simulink model "21-E"  (R2014a)
settings: Solver=FixedStepDiscrete  StartTime=0.0  StopTime=10.0  FixedStep=0.0005  RelTol=1e-3
undefined symbols (not defined in the file): add_k1_100, add_k2_100, ADDspeed, cal_acc_div, cal_acc_flo_add, cal_acc_min, cal_an_div, cal_an_min, cal_bre_div, cal_bre_en_add, cal_bre_flo_add, cal_bre_min, cal_conf_off, cal_conf_on, controller, ecucoder_acal, enres_on_add, enres_per_add
libraries: simulink x165, ec55xxlib x29
(part 4 of 6)

== system 21-E/ECU_can/ECU_sig1/yaw_r ==
  yaw_r : Inport
  Constant{1..2,4..8} (7 alike) : Constant  Value=0  OutDataTypeStr=uint8  SampleTime=-1
  yaw_rABS : Abs
  yaw_rCS : ArithShift  BitShiftNumber=-8
  yaw_rConS : Constant  OutDataTypeStr=single
  yaw_rCosR : Constant  Value=0  OutDataTypeStr=uint8
  yaw_rROP : RelationalOperator  Operator=<  OutDataTypeStr=boolean
  yaw_rRon : Rounding  Operator=round
  yaw_rSW : Switch  Criteria=u2 ~= 0
  yaw_r_1sat : Saturate  UpperLimit=255  LowerLimit=0
  yaw_r_Convert : DataTypeConversion  OutDataTypeStr=uint8
  yaw_r_Convert1 : DataTypeConversion  OutDataTypeStr=uint32
  yaw_r_D : Product  Inputs=*/
  yaw_r_F : Constant  OutDataTypeStr=single
  yaw_r_L : simulink/Logic and Bit Operations/Bitwise Operator  logicop=AND  UseBitMask=on  BitMask=255  BitMaskRealWorld=Stored Integer
  yaw_r_O : Constant  Value=0  OutDataTypeStr=single
  yaw_r_S : ArithShift
  yaw_r_sat : Saturate  UpperLimit=255  LowerLimit=0
  yaw_r_st : Sum  Inputs=+-
  yaw_rsubcon : Sum  Inputs=+-
  output1 : Outport
  output2 : Outport  Port=2
  output3 : Outport  Port=3
  output4 : Outport  Port=4
  output5 : Outport  Port=5
  output6 : Outport  Port=6
  output7 : Outport  Port=7
  output8 : Outport  Port=8
  wires:
  Constant8/1 -> output8/1
  Constant7/1 -> output7/1
  Constant6/1 -> output6/1
  Constant5/1 -> output5/1
  Constant4/1 -> output4/1
  Constant2/1 -> output2/1
  Constant1/1 -> output1/1
  yaw_r_Convert/1 -> output3/1
  yaw_r_L/1 -> yaw_r_Convert/1
  yaw_r_Convert1/1 -> yaw_r_L/1
  yaw_r_1sat/1 -> yaw_r_Convert1/1
  yaw_r_S/1 -> yaw_r_1sat/1
  yaw_rSW/1 -> yaw_r_S/1
  yaw_rROP/1 -> yaw_rSW/2
  yaw_rsubcon/1 -> yaw_rSW/1
  yaw_rABS/1 -> yaw_rsubcon/2
  yaw_rCS/1 -> yaw_rsubcon/1
  yaw_rConS/1 -> yaw_rCS/1
  yaw_rCosR/1 -> yaw_rROP/2
  yaw_rRon/1 -> yaw_rSW/3, yaw_rABS/1, yaw_rROP/1
  yaw_r_D/1 -> yaw_rRon/1
  yaw_r_F/1 -> yaw_r_D/2
  yaw_r_st/1 -> yaw_r_D/1
  yaw_r_O/1 -> yaw_r_st/2
  yaw_r_sat/1 -> yaw_r_st/1
  yaw_r/1 -> yaw_r_sat/1

== system 21-E/ECU_can/ECU_speed/v_1L ==
  v_1L : Inport
  BitCov : DataTypeConversion  OutDataTypeStr=uint8
  Constant{3..8} (6 alike) : Constant  Value=0  OutDataTypeStr=uint8
  v_1LCOV : DataTypeConversion  OutDataTypeStr=uint8
  v_1LRon : Rounding  Operator=round
  v_1L_1sat : Saturate  UpperLimit=65535  LowerLimit=0
  v_1L_And : simulink/Logic and Bit Operations/Bitwise Operator  logicop=AND  UseBitMask=off  NumInputPorts=2  BitMask=bin2dec('11011001')  BitMaskRealWorld=Stored Integer
  v_1L_And_C : Constant  Value=255  OutDataTypeStr=uint32
  v_1L_Convert : DataTypeConversion  OutDataTypeStr=uint32
  v_1L_D : Product  Inputs=*/
  v_1L_D1 : Product  Inputs=*/
  v_1L_F : Constant  OutDataTypeStr=single
  v_1L_L : simulink/Logic and Bit Operations/Bitwise Operator  logicop=AND  UseBitMask=on  BitMask=65535  BitMaskRealWorld=Stored Integer
  v_1L_O : Constant  Value=0  OutDataTypeStr=single
  v_1L_S : ArithShift
  v_1L_sat : Saturate  UpperLimit=65535  LowerLimit=0
  v_1L_st : Sum  Inputs=+-
  v_1Loutput2_C : Constant  Value=256
  output1 : Outport
  output2 : Outport  Port=2
  output3 : Outport  Port=3
  output4 : Outport  Port=4
  output5 : Outport  Port=5
  output6 : Outport  Port=6
  output7 : Outport  Port=7
  output8 : Outport  Port=8
  wires:
  Constant8/1 -> output8/1
  Constant7/1 -> output7/1
  Constant6/1 -> output6/1
  Constant5/1 -> output5/1
  Constant4/1 -> output4/1
  Constant3/1 -> output3/1
  BitCov/1 -> output1/1
  v_1L_And/1 -> BitCov/1
  v_1L_And_C/1 -> v_1L_And/2
  v_1LCOV/1 -> output2/1
  v_1L_D1/1 -> v_1LCOV/1
  v_1Loutput2_C/1 -> v_1L_D1/2
  v_1L_L/1 -> v_1L_And/1, v_1L_D1/1
  v_1L_Convert/1 -> v_1L_L/1
  v_1L_1sat/1 -> v_1L_Convert/1
  v_1L_S/1 -> v_1L_1sat/1
  v_1LRon/1 -> v_1L_S/1
  v_1L_D/1 -> v_1LRon/1
  v_1L_F/1 -> v_1L_D/2
  v_1L_st/1 -> v_1L_D/1
  v_1L_O/1 -> v_1L_st/2
  v_1L_sat/1 -> v_1L_st/1
  v_1L/1 -> v_1L_sat/1

== system 21-E/ECU_can/ECU_speed/v_1R ==
  v_1R : Inport
  BitCov : DataTypeConversion  OutDataTypeStr=uint8
  Constant{1..2,5..8} (6 alike) : Constant  Value=0  OutDataTypeStr=uint8
  v_1RCOV : DataTypeConversion  OutDataTypeStr=uint8
  v_1RRon : Rounding  Operator=round
  v_1R_1sat : Saturate  UpperLimit=65535  LowerLimit=0
  v_1R_And : simulink/Logic and Bit Operations/Bitwise Operator  logicop=AND  UseBitMask=off  NumInputPorts=2  BitMask=bin2dec('11011001')  BitMaskRealWorld=Stored Integer
  v_1R_And_C : Constant  Value=255  OutDataTypeStr=uint32
  v_1R_Convert : DataTypeConversion  OutDataTypeStr=uint32
  v_1R_D : Product  Inputs=*/
  v_1R_D1 : Product  Inputs=*/
  v_1R_F : Constant  OutDataTypeStr=single
  v_1R_L : simulink/Logic and Bit Operations/Bitwise Operator  logicop=AND  UseBitMask=on  BitMask=65535  BitMaskRealWorld=Stored Integer
  v_1R_O : Constant  Value=0  OutDataTypeStr=single
  v_1R_S : ArithShift
  v_1R_sat : Saturate  UpperLimit=65535  LowerLimit=0
  v_1R_st : Sum  Inputs=+-
  v_1Routput4_C : Constant  Value=256
  output1 : Outport
  output2 : Outport  Port=2
  output3 : Outport  Port=3
  output4 : Outport  Port=4
  output5 : Outport  Port=5
  output6 : Outport  Port=6
  output7 : Outport  Port=7
  output8 : Outport  Port=8
  wires:
  Constant8/1 -> output8/1
  Constant7/1 -> output7/1
  Constant6/1 -> output6/1
  Constant5/1 -> output5/1
  Constant2/1 -> output2/1
  Constant1/1 -> output1/1
  BitCov/1 -> output3/1
  v_1R_And/1 -> BitCov/1
  v_1R_And_C/1 -> v_1R_And/2
  v_1RCOV/1 -> output4/1
  v_1R_D1/1 -> v_1RCOV/1
  v_1Routput4_C/1 -> v_1R_D1/2
  v_1R_L/1 -> v_1R_And/1, v_1R_D1/1
  v_1R_Convert/1 -> v_1R_L/1
  v_1R_1sat/1 -> v_1R_Convert/1
  v_1R_S/1 -> v_1R_1sat/1
  v_1RRon/1 -> v_1R_S/1
  v_1R_D/1 -> v_1RRon/1
  v_1R_F/1 -> v_1R_D/2
  v_1R_st/1 -> v_1R_D/1
  v_1R_O/1 -> v_1R_st/2
  v_1R_sat/1 -> v_1R_st/1
  v_1R/1 -> v_1R_sat/1

== system 21-E/ECU_can/ECU_speed/v_2L ==
  v_2L : Inport
  BitCov : DataTypeConversion  OutDataTypeStr=uint8
  Constant{1..4,7..8} (6 alike) : Constant  Value=0  OutDataTypeStr=uint8
  v_2LCOV : DataTypeConversion  OutDataTypeStr=uint8
  v_2LRon : Rounding  Operator=round
  v_2L_1sat : Saturate  UpperLimit=65535  LowerLimit=0
  v_2L_And : simulink/Logic and Bit Operations/Bitwise Operator  logicop=AND  UseBitMask=off  NumInputPorts=2  BitMask=bin2dec('11011001')  BitMaskRealWorld=Stored Integer
  v_2L_And_C : Constant  Value=255  OutDataTypeStr=uint32
  v_2L_Convert : DataTypeConversion  OutDataTypeStr=uint32
  v_2L_D : Product  Inputs=*/
  v_2L_D1 : Product  Inputs=*/
  v_2L_F : Constant  OutDataTypeStr=single
  v_2L_L : simulink/Logic and Bit Operations/Bitwise Operator  logicop=AND  UseBitMask=on  BitMask=65535  BitMaskRealWorld=Stored Integer
  v_2L_O : Constant  Value=0  OutDataTypeStr=single
  v_2L_S : ArithShift
  v_2L_sat : Saturate  UpperLimit=65535  LowerLimit=0
  v_2L_st : Sum  Inputs=+-
  v_2Loutput6_C : Constant  Value=256
  output1 : Outport
  output2 : Outport  Port=2
  output3 : Outport  Port=3
  output4 : Outport  Port=4
  output5 : Outport  Port=5
  output6 : Outport  Port=6
  output7 : Outport  Port=7
  output8 : Outport  Port=8
  wires:
  Constant8/1 -> output8/1
  Constant7/1 -> output7/1
  Constant4/1 -> output4/1
  Constant3/1 -> output3/1
  Constant2/1 -> output2/1
  Constant1/1 -> output1/1
  BitCov/1 -> output5/1
  v_2L_And/1 -> BitCov/1
  v_2L_And_C/1 -> v_2L_And/2
  v_2LCOV/1 -> output6/1
  v_2L_D1/1 -> v_2LCOV/1
  v_2Loutput6_C/1 -> v_2L_D1/2
  v_2L_L/1 -> v_2L_And/1, v_2L_D1/1
  v_2L_Convert/1 -> v_2L_L/1
  v_2L_1sat/1 -> v_2L_Convert/1
  v_2L_S/1 -> v_2L_1sat/1
  v_2LRon/1 -> v_2L_S/1
  v_2L_D/1 -> v_2LRon/1
  v_2L_F/1 -> v_2L_D/2
  v_2L_st/1 -> v_2L_D/1
  v_2L_O/1 -> v_2L_st/2
  v_2L_sat/1 -> v_2L_st/1
  v_2L/1 -> v_2L_sat/1

== system 21-E/ECU_can/ECU_speed/v_2R ==
  v_2R : Inport
  BitCov : DataTypeConversion  OutDataTypeStr=uint8
  Constant{1..6} (6 alike) : Constant  Value=0  OutDataTypeStr=uint8
  v_2RCOV : DataTypeConversion  OutDataTypeStr=uint8
  v_2RRon : Rounding  Operator=round
  v_2R_1sat : Saturate  UpperLimit=65535  LowerLimit=0
  v_2R_And : simulink/Logic and Bit Operations/Bitwise Operator  logicop=AND  UseBitMask=off  NumInputPorts=2  BitMask=bin2dec('11011001')  BitMaskRealWorld=Stored Integer
  v_2R_And_C : Constant  Value=255  OutDataTypeStr=uint32
  v_2R_Convert : DataTypeConversion  OutDataTypeStr=uint32
  v_2R_D : Product  Inputs=*/
  v_2R_D1 : Product  Inputs=*/
  v_2R_F : Constant  OutDataTypeStr=single
  v_2R_L : simulink/Logic and Bit Operations/Bitwise Operator  logicop=AND  UseBitMask=on  BitMask=65535  BitMaskRealWorld=Stored Integer
  v_2R_O : Constant  Value=0  OutDataTypeStr=single
  v_2R_S : ArithShift
  v_2R_sat : Saturate  UpperLimit=65535  LowerLimit=0
  v_2R_st : Sum  Inputs=+-
  v_2Routput8_C : Constant  Value=256
  output1 : Outport
  output2 : Outport  Port=2
  output3 : Outport  Port=3
  output4 : Outport  Port=4
  output5 : Outport  Port=5
  output6 : Outport  Port=6
  output7 : Outport  Port=7
  output8 : Outport  Port=8
  wires:
  Constant6/1 -> output6/1
  Constant5/1 -> output5/1
  Constant4/1 -> output4/1
  Constant3/1 -> output3/1
  Constant2/1 -> output2/1
  Constant1/1 -> output1/1
  BitCov/1 -> output7/1
  v_2R_And/1 -> BitCov/1
  v_2R_And_C/1 -> v_2R_And/2
  v_2RCOV/1 -> output8/1
  v_2R_D1/1 -> v_2RCOV/1
  v_2Routput8_C/1 -> v_2R_D1/2
  v_2R_L/1 -> v_2R_And/1, v_2R_D1/1
  v_2R_Convert/1 -> v_2R_L/1
  v_2R_1sat/1 -> v_2R_Convert/1
  v_2R_S/1 -> v_2R_1sat/1
  v_2RRon/1 -> v_2R_S/1
  v_2R_D/1 -> v_2RRon/1
  v_2R_F/1 -> v_2R_D/2
  v_2R_st/1 -> v_2R_D/1
  v_2R_O/1 -> v_2R_st/2
  v_2R_sat/1 -> v_2R_st/1
  v_2R/1 -> v_2R_sat/1

== system 21-E/ECU_can/ECU_tem/IGBT_1 ==
  IGBT_1 : Inport
  Constant{2..8} (7 alike) : Constant  Value=0  OutDataTypeStr=uint8
  IGBT_1Ron : Rounding  Operator=round
  IGBT_1_1sat : Saturate  UpperLimit=255  LowerLimit=0
  IGBT_1_Convert : DataTypeConversion  OutDataTypeStr=uint8
  IGBT_1_Convert1 : DataTypeConversion  OutDataTypeStr=uint32
  IGBT_1_D : Product  Inputs=*/
  IGBT_1_F : Constant  OutDataTypeStr=single
  IGBT_1_L : simulink/Logic and Bit Operations/Bitwise Operator  logicop=AND  UseBitMask=on  BitMask=255  BitMaskRealWorld=Stored Integer
  IGBT_1_O : Constant  Value=0  OutDataTypeStr=single
  IGBT_1_S : ArithShift
  IGBT_1_sat : Saturate  UpperLimit=255  LowerLimit=0
  IGBT_1_st : Sum  Inputs=+-
  output1 : Outport
  output2 : Outport  Port=2
  output3 : Outport  Port=3
  output4 : Outport  Port=4
  output5 : Outport  Port=5
  output6 : Outport  Port=6
  output7 : Outport  Port=7
  output8 : Outport  Port=8
  wires:
  Constant8/1 -> output8/1
  Constant7/1 -> output7/1
  Constant6/1 -> output6/1
  Constant5/1 -> output5/1
  Constant4/1 -> output4/1
  Constant3/1 -> output3/1
  Constant2/1 -> output2/1
  IGBT_1_Convert/1 -> output1/1
  IGBT_1_L/1 -> IGBT_1_Convert/1
  IGBT_1_Convert1/1 -> IGBT_1_L/1
  IGBT_1_1sat/1 -> IGBT_1_Convert1/1
  IGBT_1_S/1 -> IGBT_1_1sat/1
  IGBT_1Ron/1 -> IGBT_1_S/1
  IGBT_1_D/1 -> IGBT_1Ron/1
  IGBT_1_F/1 -> IGBT_1_D/2
  IGBT_1_st/1 -> IGBT_1_D/1
  IGBT_1_O/1 -> IGBT_1_st/2
  IGBT_1_sat/1 -> IGBT_1_st/1
  IGBT_1/1 -> IGBT_1_sat/1

== system 21-E/ECU_can/ECU_tem/IGBT_2 ==
  IGBT_2 : Inport
  Constant{1,3..8} (7 alike) : Constant  Value=0  OutDataTypeStr=uint8
  IGBT_2Ron : Rounding  Operator=round
  IGBT_2_1sat : Saturate  UpperLimit=255  LowerLimit=0
  IGBT_2_Convert : DataTypeConversion  OutDataTypeStr=uint8
  IGBT_2_Convert1 : DataTypeConversion  OutDataTypeStr=uint32
  IGBT_2_D : Product  Inputs=*/
  IGBT_2_F : Constant  OutDataTypeStr=single
  IGBT_2_L : simulink/Logic and Bit Operations/Bitwise Operator  logicop=AND  UseBitMask=on  BitMask=255  BitMaskRealWorld=Stored Integer
  IGBT_2_O : Constant  Value=0  OutDataTypeStr=single
  IGBT_2_S : ArithShift
  IGBT_2_sat : Saturate  UpperLimit=255  LowerLimit=0
  IGBT_2_st : Sum  Inputs=+-
  output1 : Outport
  output2 : Outport  Port=2
  output3 : Outport  Port=3
  output4 : Outport  Port=4
  output5 : Outport  Port=5
  output6 : Outport  Port=6
  output7 : Outport  Port=7
  output8 : Outport  Port=8
  wires:
  Constant8/1 -> output8/1
  Constant7/1 -> output7/1
  Constant6/1 -> output6/1
  Constant5/1 -> output5/1
  Constant4/1 -> output4/1
  Constant3/1 -> output3/1
  Constant1/1 -> output1/1
  IGBT_2_Convert/1 -> output2/1
  IGBT_2_L/1 -> IGBT_2_Convert/1
  IGBT_2_Convert1/1 -> IGBT_2_L/1
  IGBT_2_1sat/1 -> IGBT_2_Convert1/1
  IGBT_2_S/1 -> IGBT_2_1sat/1
  IGBT_2Ron/1 -> IGBT_2_S/1
  IGBT_2_D/1 -> IGBT_2Ron/1
  IGBT_2_F/1 -> IGBT_2_D/2
  IGBT_2_st/1 -> IGBT_2_D/1
  IGBT_2_O/1 -> IGBT_2_st/2
  IGBT_2_sat/1 -> IGBT_2_st/1
  IGBT_2/1 -> IGBT_2_sat/1

== system 21-E/ECU_can/ECU_tem/IGBT_3 ==
  IGBT_3 : Inport
  Constant{1..2,4..8} (7 alike) : Constant  Value=0  OutDataTypeStr=uint8
  IGBT_3Ron : Rounding  Operator=round
  IGBT_3_1sat : Saturate  UpperLimit=255  LowerLimit=0
  IGBT_3_Convert : DataTypeConversion  OutDataTypeStr=uint8
  IGBT_3_Convert1 : DataTypeConversion  OutDataTypeStr=uint32
  IGBT_3_D : Product  Inputs=*/
  IGBT_3_F : Constant  OutDataTypeStr=single
  IGBT_3_L : simulink/Logic and Bit Operations/Bitwise Operator  logicop=AND  UseBitMask=on  BitMask=255  BitMaskRealWorld=Stored Integer
  IGBT_3_O : Constant  Value=0  OutDataTypeStr=single
  IGBT_3_S : ArithShift
  IGBT_3_sat : Saturate  UpperLimit=255  LowerLimit=0
  IGBT_3_st : Sum  Inputs=+-
  output1 : Outport
  output2 : Outport  Port=2
  output3 : Outport  Port=3
  output4 : Outport  Port=4
  output5 : Outport  Port=5
  output6 : Outport  Port=6
  output7 : Outport  Port=7
  output8 : Outport  Port=8
  wires:
  Constant8/1 -> output8/1
  Constant7/1 -> output7/1
  Constant6/1 -> output6/1
  Constant5/1 -> output5/1
  Constant4/1 -> output4/1
  Constant2/1 -> output2/1
  Constant1/1 -> output1/1
  IGBT_3_Convert/1 -> output3/1
  IGBT_3_L/1 -> IGBT_3_Convert/1
  IGBT_3_Convert1/1 -> IGBT_3_L/1
  IGBT_3_1sat/1 -> IGBT_3_Convert1/1
  IGBT_3_S/1 -> IGBT_3_1sat/1
  IGBT_3Ron/1 -> IGBT_3_S/1
  IGBT_3_D/1 -> IGBT_3Ron/1
  IGBT_3_F/1 -> IGBT_3_D/2
  IGBT_3_st/1 -> IGBT_3_D/1
  IGBT_3_O/1 -> IGBT_3_st/2
  IGBT_3_sat/1 -> IGBT_3_st/1
  IGBT_3/1 -> IGBT_3_sat/1

== system 21-E/ECU_can/ECU_tem/IGBT_4 ==
  IGBT_4 : Inport
  Constant{1..3,5..8} (7 alike) : Constant  Value=0  OutDataTypeStr=uint8
  IGBT_4Ron : Rounding  Operator=round
  IGBT_4_1sat : Saturate  UpperLimit=255  LowerLimit=0
  IGBT_4_Convert : DataTypeConversion  OutDataTypeStr=uint8
  IGBT_4_Convert1 : DataTypeConversion  OutDataTypeStr=uint32
  IGBT_4_D : Product  Inputs=*/
  IGBT_4_F : Constant  OutDataTypeStr=single
  IGBT_4_L : simulink/Logic and Bit Operations/Bitwise Operator  logicop=AND  UseBitMask=on  BitMask=255  BitMaskRealWorld=Stored Integer
  IGBT_4_O : Constant  Value=0  OutDataTypeStr=single
  IGBT_4_S : ArithShift
  IGBT_4_sat : Saturate  UpperLimit=255  LowerLimit=0
  IGBT_4_st : Sum  Inputs=+-
  output1 : Outport
  output2 : Outport  Port=2
  output3 : Outport  Port=3
  output4 : Outport  Port=4
  output5 : Outport  Port=5
  output6 : Outport  Port=6
  output7 : Outport  Port=7
  output8 : Outport  Port=8
  wires:
  Constant8/1 -> output8/1
  Constant7/1 -> output7/1
  Constant6/1 -> output6/1
  Constant5/1 -> output5/1
  Constant3/1 -> output3/1
  Constant2/1 -> output2/1
  Constant1/1 -> output1/1
  IGBT_4_Convert/1 -> output4/1
  IGBT_4_L/1 -> IGBT_4_Convert/1
  IGBT_4_Convert1/1 -> IGBT_4_L/1
  IGBT_4_1sat/1 -> IGBT_4_Convert1/1
  IGBT_4_S/1 -> IGBT_4_1sat/1
  IGBT_4Ron/1 -> IGBT_4_S/1
  IGBT_4_D/1 -> IGBT_4Ron/1
  IGBT_4_F/1 -> IGBT_4_D/2
  IGBT_4_st/1 -> IGBT_4_D/1
  IGBT_4_O/1 -> IGBT_4_st/2
  IGBT_4_sat/1 -> IGBT_4_st/1
  IGBT_4/1 -> IGBT_4_sat/1

== system 21-E/ECU_can/ECU_tem/Mot_1 ==
  Mot_1 : Inport
  Constant{1..4,6..8} (7 alike) : Constant  Value=0  OutDataTypeStr=uint8
  Mot_1Ron : Rounding  Operator=round
  Mot_1_1sat : Saturate  UpperLimit=255  LowerLimit=0
  Mot_1_Convert : DataTypeConversion  OutDataTypeStr=uint8
  Mot_1_Convert1 : DataTypeConversion  OutDataTypeStr=uint32
  Mot_1_D : Product  Inputs=*/
  Mot_1_F : Constant  OutDataTypeStr=single
  Mot_1_L : simulink/Logic and Bit Operations/Bitwise Operator  logicop=AND  UseBitMask=on  BitMask=255  BitMaskRealWorld=Stored Integer
  Mot_1_O : Constant  Value=0  OutDataTypeStr=single
  Mot_1_S : ArithShift
  Mot_1_sat : Saturate  UpperLimit=255  LowerLimit=0
  Mot_1_st : Sum  Inputs=+-
  output1 : Outport
  output2 : Outport  Port=2
  output3 : Outport  Port=3
  output4 : Outport  Port=4
  output5 : Outport  Port=5
  output6 : Outport  Port=6
  output7 : Outport  Port=7
  output8 : Outport  Port=8
  wires:
  Constant8/1 -> output8/1
  Constant7/1 -> output7/1
  Constant6/1 -> output6/1
  Constant4/1 -> output4/1
  Constant3/1 -> output3/1
  Constant2/1 -> output2/1
  Constant1/1 -> output1/1
  Mot_1_Convert/1 -> output5/1
  Mot_1_L/1 -> Mot_1_Convert/1
  Mot_1_Convert1/1 -> Mot_1_L/1
  Mot_1_1sat/1 -> Mot_1_Convert1/1
  Mot_1_S/1 -> Mot_1_1sat/1
  Mot_1Ron/1 -> Mot_1_S/1
  Mot_1_D/1 -> Mot_1Ron/1
  Mot_1_F/1 -> Mot_1_D/2
  Mot_1_st/1 -> Mot_1_D/1
  Mot_1_O/1 -> Mot_1_st/2
  Mot_1_sat/1 -> Mot_1_st/1
  Mot_1/1 -> Mot_1_sat/1

== system 21-E/ECU_can/ECU_tem/Mot_2 ==
  Mot_2 : Inport
  Constant{1..5,7..8} (7 alike) : Constant  Value=0  OutDataTypeStr=uint8
  Mot_2Ron : Rounding  Operator=round
  Mot_2_1sat : Saturate  UpperLimit=255  LowerLimit=0
  Mot_2_Convert : DataTypeConversion  OutDataTypeStr=uint8
  Mot_2_Convert1 : DataTypeConversion  OutDataTypeStr=uint32
  Mot_2_D : Product  Inputs=*/
  Mot_2_F : Constant  OutDataTypeStr=single
  Mot_2_L : simulink/Logic and Bit Operations/Bitwise Operator  logicop=AND  UseBitMask=on  BitMask=255  BitMaskRealWorld=Stored Integer
  Mot_2_O : Constant  Value=0  OutDataTypeStr=single
  Mot_2_S : ArithShift
  Mot_2_sat : Saturate  UpperLimit=255  LowerLimit=0
  Mot_2_st : Sum  Inputs=+-
  output1 : Outport
  output2 : Outport  Port=2
  output3 : Outport  Port=3
  output4 : Outport  Port=4
  output5 : Outport  Port=5
  output6 : Outport  Port=6
  output7 : Outport  Port=7
  output8 : Outport  Port=8
  wires:
  Constant8/1 -> output8/1
  Constant7/1 -> output7/1
  Constant5/1 -> output5/1
  Constant4/1 -> output4/1
  Constant3/1 -> output3/1
  Constant2/1 -> output2/1
  Constant1/1 -> output1/1
  Mot_2_Convert/1 -> output6/1
  Mot_2_L/1 -> Mot_2_Convert/1
  Mot_2_Convert1/1 -> Mot_2_L/1
  Mot_2_1sat/1 -> Mot_2_Convert1/1
  Mot_2_S/1 -> Mot_2_1sat/1
  Mot_2Ron/1 -> Mot_2_S/1
  Mot_2_D/1 -> Mot_2Ron/1
  Mot_2_F/1 -> Mot_2_D/2
  Mot_2_st/1 -> Mot_2_D/1
  Mot_2_O/1 -> Mot_2_st/2
  Mot_2_sat/1 -> Mot_2_st/1
  Mot_2/1 -> Mot_2_sat/1

== system 21-E/ECU_can/ECU_tem/Mot_3 ==
  Mot_3 : Inport
  Constant{1..6,8} (7 alike) : Constant  Value=0  OutDataTypeStr=uint8
  Mot_3Ron : Rounding  Operator=round
  Mot_3_1sat : Saturate  UpperLimit=255  LowerLimit=0
  Mot_3_Convert : DataTypeConversion  OutDataTypeStr=uint8
  Mot_3_Convert1 : DataTypeConversion  OutDataTypeStr=uint32
  Mot_3_D : Product  Inputs=*/
  Mot_3_F : Constant  OutDataTypeStr=single
  Mot_3_L : simulink/Logic and Bit Operations/Bitwise Operator  logicop=AND  UseBitMask=on  BitMask=255  BitMaskRealWorld=Stored Integer
  Mot_3_O : Constant  Value=0  OutDataTypeStr=single
  Mot_3_S : ArithShift
  Mot_3_sat : Saturate  UpperLimit=255  LowerLimit=0
  Mot_3_st : Sum  Inputs=+-
  output1 : Outport
  output2 : Outport  Port=2
  output3 : Outport  Port=3
  output4 : Outport  Port=4
  output5 : Outport  Port=5
  output6 : Outport  Port=6
  output7 : Outport  Port=7
  output8 : Outport  Port=8
  wires:
  Constant8/1 -> output8/1
  Constant6/1 -> output6/1
  Constant5/1 -> output5/1
  Constant4/1 -> output4/1
  Constant3/1 -> output3/1
  Constant2/1 -> output2/1
  Constant1/1 -> output1/1
  Mot_3_Convert/1 -> output7/1
  Mot_3_L/1 -> Mot_3_Convert/1
  Mot_3_Convert1/1 -> Mot_3_L/1
  Mot_3_1sat/1 -> Mot_3_Convert1/1
  Mot_3_S/1 -> Mot_3_1sat/1
  Mot_3Ron/1 -> Mot_3_S/1
  Mot_3_D/1 -> Mot_3Ron/1
  Mot_3_F/1 -> Mot_3_D/2
  Mot_3_st/1 -> Mot_3_D/1
  Mot_3_O/1 -> Mot_3_st/2
  Mot_3_sat/1 -> Mot_3_st/1
  Mot_3/1 -> Mot_3_sat/1

== system 21-E/ECU_can/ECU_tem/Mot_4 ==
  Mot_4 : Inport
  Constant{1..7} (7 alike) : Constant  Value=0  OutDataTypeStr=uint8
  Mot_4Ron : Rounding  Operator=round
  Mot_4_1sat : Saturate  UpperLimit=255  LowerLimit=0
  Mot_4_Convert : DataTypeConversion  OutDataTypeStr=uint8
  Mot_4_Convert1 : DataTypeConversion  OutDataTypeStr=uint32
  Mot_4_D : Product  Inputs=*/
  Mot_4_F : Constant  OutDataTypeStr=single
  Mot_4_L : simulink/Logic and Bit Operations/Bitwise Operator  logicop=AND  UseBitMask=on  BitMask=255  BitMaskRealWorld=Stored Integer
  Mot_4_O : Constant  Value=0  OutDataTypeStr=single
  Mot_4_S : ArithShift
  Mot_4_sat : Saturate  UpperLimit=255  LowerLimit=0
  Mot_4_st : Sum  Inputs=+-
  output1 : Outport
  output2 : Outport  Port=2
  output3 : Outport  Port=3
  output4 : Outport  Port=4
  output5 : Outport  Port=5
  output6 : Outport  Port=6
  output7 : Outport  Port=7
  output8 : Outport  Port=8
  wires:
  Constant7/1 -> output7/1
  Constant6/1 -> output6/1
  Constant5/1 -> output5/1
  Constant4/1 -> output4/1
  Constant3/1 -> output3/1
  Constant2/1 -> output2/1
  Constant1/1 -> output1/1
  Mot_4_Convert/1 -> output8/1
  Mot_4_L/1 -> Mot_4_Convert/1
  Mot_4_Convert1/1 -> Mot_4_L/1
  Mot_4_1sat/1 -> Mot_4_Convert1/1
  Mot_4_S/1 -> Mot_4_1sat/1
  Mot_4Ron/1 -> Mot_4_S/1
  Mot_4_D/1 -> Mot_4Ron/1
  Mot_4_F/1 -> Mot_4_D/2
  Mot_4_st/1 -> Mot_4_D/1
  Mot_4_O/1 -> Mot_4_st/2
  Mot_4_sat/1 -> Mot_4_st/1
  Mot_4/1 -> Mot_4_sat/1

== system 21-E/angle/angle2/angle_1_Sub ==
  In1 : Inport
  Out1 : Outport
  wires:
  In1/1 -> Out1/1

== system 21-E/angle/angle2/angle_2_Sub ==
  In1 : Inport
  Out1 : Outport
  wires:
  In1/1 -> Out1/1

== system 21-E/angle/angle2/un_1_Sub ==
  In1 : Inport
  Out1 : Outport
  wires:
  In1/1 -> Out1/1

== system 21-E/angle/angle2/un_2_Sub ==
  In1 : Inport
  Out1 : Outport
  wires:
  In1/1 -> Out1/1

== system 21-E/angle/angle2/un_3_Sub ==
  In1 : Inport
  Out1 : Outport
  wires:
  In1/1 -> Out1/1

== system 21-E/mot_trans/AMK_dyn_1L/MI_1L_Sub ==
  In1 : Inport
  Out1 : Outport
  wires:
  In1/1 -> Out1/1

== system 21-E/mot_trans/AMK_dyn_1L/TI_1L_Sub ==
  In1 : Inport
  Out1 : Outport
  wires:
  In1/1 -> Out1/1

== system 21-E/mot_trans/AMK_dyn_1L/s_1L_Sub ==
  In1 : Inport
  Out1 : Outport
  wires:
  In1/1 -> Out1/1

== system 21-E/mot_trans/AMK_dyn_1L/v_1L_Sub ==
  In1 : Inport
  Out1 : Outport
  wires:
  In1/1 -> Out1/1

== system 21-E/mot_trans/AMK_dyn_1R/MI_1R_Sub ==
  In1 : Inport
  Out1 : Outport
  wires:
  In1/1 -> Out1/1

== system 21-E/mot_trans/AMK_dyn_1R/TI_1R_Sub ==
  In1 : Inport
  Out1 : Outport
  wires:
  In1/1 -> Out1/1

== system 21-E/mot_trans/AMK_dyn_1R/s_1R_Sub ==
  In1 : Inport
  Out1 : Outport
  wires:
  In1/1 -> Out1/1

== system 21-E/mot_trans/AMK_dyn_1R/v_1R_Sub ==
  In1 : Inport
  Out1 : Outport
  wires:
  In1/1 -> Out1/1

== system 21-E/mot_trans/AMK_dyn_2L/MI_2L_Sub ==
  In1 : Inport
  Out1 : Outport
  wires:
  In1/1 -> Out1/1

== system 21-E/mot_trans/AMK_dyn_2L/TI_2L_Sub ==
  In1 : Inport
  Out1 : Outport
  wires:
  In1/1 -> Out1/1

== system 21-E/mot_trans/AMK_dyn_2L/s_2L_Sub ==
  In1 : Inport
  Out1 : Outport
  wires:
  In1/1 -> Out1/1

== system 21-E/mot_trans/AMK_dyn_2L/v_2L_Sub ==
  In1 : Inport
  Out1 : Outport
  wires:
  In1/1 -> Out1/1

== system 21-E/mot_trans/AMK_dyn_2R/MI_2R_Sub ==
  In1 : Inport
  Out1 : Outport
  wires:
  In1/1 -> Out1/1

== system 21-E/mot_trans/AMK_dyn_2R/TI_2R_Sub ==
  In1 : Inport
  Out1 : Outport
  wires:
  In1/1 -> Out1/1

== system 21-E/mot_trans/AMK_dyn_2R/s_2R_Sub ==
  In1 : Inport
  Out1 : Outport
  wires:
  In1/1 -> Out1/1

== system 21-E/mot_trans/AMK_dyn_2R/v_2R_Sub ==
  In1 : Inport
  Out1 : Outport
  wires:
  In1/1 -> Out1/1

== system 21-E/mot_trans/AMK_tem_1L/IGBT_1L_Sub ==
  In1 : Inport
  Out1 : Outport
  wires:
  In1/1 -> Out1/1

== system 21-E/mot_trans/AMK_tem_1L/Inv_1L_Sub ==
  In1 : Inport
  Out1 : Outport
  wires:
  In1/1 -> Out1/1

== system 21-E/mot_trans/AMK_tem_1L/Mot_1L_Sub ==
  In1 : Inport
  Out1 : Outport
  wires:
  In1/1 -> Out1/1

== system 21-E/mot_trans/AMK_tem_1L/error_1L_Sub ==
  In1 : Inport
  Out1 : Outport
  wires:
  In1/1 -> Out1/1

== system 21-E/mot_trans/AMK_tem_1R/IGBT_1R_Sub ==
  In1 : Inport
  Out1 : Outport
  wires:
  In1/1 -> Out1/1

== system 21-E/mot_trans/AMK_tem_1R/Inv_1R_Sub ==
  In1 : Inport
  Out1 : Outport
  wires:
  In1/1 -> Out1/1

== system 21-E/mot_trans/AMK_tem_1R/Mot_1R_Sub ==
  In1 : Inport
  Out1 : Outport
  wires:
  In1/1 -> Out1/1

== system 21-E/mot_trans/AMK_tem_1R/error_1R_Sub ==
  In1 : Inport
  Out1 : Outport
  wires:
  In1/1 -> Out1/1

== system 21-E/mot_trans/AMK_tem_2L/IGBT_2L_Sub ==
  In1 : Inport
  Out1 : Outport
  wires:
  In1/1 -> Out1/1

== system 21-E/mot_trans/AMK_tem_2L/Inv_2L_Sub ==
  In1 : Inport
  Out1 : Outport
  wires:
  In1/1 -> Out1/1

== system 21-E/mot_trans/AMK_tem_2L/Mot_2L_Sub ==
  In1 : Inport
  Out1 : Outport
  wires:
  In1/1 -> Out1/1

== system 21-E/mot_trans/AMK_tem_2L/error_2L_Sub ==
  In1 : Inport
  Out1 : Outport
  wires:
  In1/1 -> Out1/1

== system 21-E/mot_trans/AMK_tem_2R/IGBT_2R_Sub ==
  In1 : Inport
  Out1 : Outport
  wires:
  In1/1 -> Out1/1

== system 21-E/mot_trans/AMK_tem_2R/Inv_2R_Sub ==
  In1 : Inport
  Out1 : Outport
  wires:
  In1/1 -> Out1/1

== system 21-E/mot_trans/AMK_tem_2R/Mot_2R_Sub ==
  In1 : Inport
  Out1 : Outport
  wires:
  In1/1 -> Out1/1

== system 21-E/mot_trans/AMK_tem_2R/error_2R_Sub ==
  In1 : Inport
  Out1 : Outport
  wires:
  In1/1 -> Out1/1

== system 21-E/run/analog_acq/jud_acc ==
  In1 : Inport
  Constant : Constant  Value=5000  OutDataTypeStr=uint16
  Constant11 : Constant  Value=100  OutDataTypeStr=uint16
  ECCalVar5 : Constant  InitFcn=ecucoder_acal;  Value=cal_acc_flo_add  OutDataTypeStr=Inherit: Inherit via back propagation  SampleTime=-1
  Logical Operator : Logic  Operator=OR  AllPortsSameDT=off  OutDataTypeStr=boolean
  Relational : RelationalOperator  Operator=<  OutDataTypeStr=boolean
  Relational Operator1 : RelationalOperator  Operator=>  OutDataTypeStr=boolean
  Sum4 : Sum  Inputs=|++
  Out1 : Outport
  wires:
  Relational/1 -> Logical Operator/2
  Logical Operator/1 -> Out1/1
  Constant/1 -> Relational Operator1/2
  Relational Operator1/1 -> Logical Operator/1
  In1/1 -> Relational Operator1/1, Relational/1
  Sum4/1 -> Relational/2
  Constant11/1 -> Sum4/1
  ECCalVar5/1 -> Sum4/2

== system 21-E/run/analog_acq/jud_bre ==
  In1 : Inport
  Constant : Constant  Value=5000  OutDataTypeStr=uint16
  Constant11 : Constant  Value=100  OutDataTypeStr=uint16
  ECCalVar5 : Constant  InitFcn=ecucoder_acal;  Value=cal_bre_flo_add  OutDataTypeStr=Inherit: Inherit via back propagation  SampleTime=-1
  Logical Operator : Logic  Operator=OR  AllPortsSameDT=off  OutDataTypeStr=boolean
  Relational Operator : RelationalOperator  Operator=<  OutDataTypeStr=boolean
  Relational Operator1 : RelationalOperator  Operator=>  OutDataTypeStr=boolean
  Sum4 : Sum  Inputs=|++
  Out1 : Outport
  wires:
  Relational Operator1/1 -> Logical Operator/1
  In1/1 -> Relational Operator/1, Relational Operator1/1
  Constant/1 -> Relational Operator1/2
  Relational Operator/1 -> Logical Operator/2
  Logical Operator/1 -> Out1/1
  Sum4/1 -> Relational Operator/2
  Constant11/1 -> Sum4/1
  ECCalVar5/1 -> Sum4/2

== system 21-E/run/cal&con/can_conf ==
  Enable : EnablePort
  Constant : Constant  Value=0  OutDataTypeStr=boolean
  Data Store Write : DataStoreWrite  DataStoreName=pedal_con
  wires:
  Constant/1 -> Data Store Write/1

== system 21-E/run/cal&con/conf ==
  Enable : EnablePort
  Constant : Constant  OutDataTypeStr=boolean
  Data Store Write : DataStoreWrite  DataStoreName=pedal_con
  wires:
  Constant/1 -> Data Store Write/1

== system 21-E/run/ctrl/ECU_1L ==
  TN_1L_in : Inport
  TP_1L_in : Inport  Port=2
  max_n_in : Inport  Port=3
  ctrl_1L_in : Inport  Port=4
  Conv{1..8} (8 alike) : DataTypeConversion
  ECU_1L_DLC : Constant  Value=8  OutDataTypeStr=uint8
  ECU_1L_DLC_Out : Terminator
  ECU_1L_ID : Constant  Value=388  OutDataTypeStr=single
  ECU_1L_ID_Out : Terminator
  ECU_1L_mux : Mux  Inputs=8
  TN_1L : Subsystem
  TP_1L : Subsystem
  ctrl_1L : Subsystem
  max_n : Subsystem
  or{1..8} (8 alike) : simulink/Logic and Bit Operations/Bitwise Operator  logicop=OR  UseBitMask=off  NumInputPorts=4  BitMask=bin2dec('11011001')  BitMaskRealWorld=Stored Integer
  output : Outport
  wires:
  ctrl_1L_in/1 -> ctrl_1L/1(ctrl_1L)
  max_n_in/1 -> max_n/1(max_n)
  TP_1L_in/1 -> TP_1L/1(TP_1L)
  TN_1L_in/1 -> TN_1L/1(TN_1L)
  ECU_1L_DLC/1 -> ECU_1L_DLC_Out/1
  ECU_1L_ID/1 -> ECU_1L_ID_Out/1
  Conv8/1 -> ECU_1L_mux/8
  or8/1 -> Conv8/1
  Conv7/1 -> ECU_1L_mux/7
  or7/1 -> Conv7/1
  Conv6/1 -> ECU_1L_mux/6
  or6/1 -> Conv6/1
  Conv5/1 -> ECU_1L_mux/5
  or5/1 -> Conv5/1
  Conv4/1 -> ECU_1L_mux/4
  or4/1 -> Conv4/1
  Conv3/1 -> ECU_1L_mux/3
  or3/1 -> Conv3/1
  Conv2/1 -> ECU_1L_mux/2
  or2/1 -> Conv2/1
  Conv1/1 -> ECU_1L_mux/1
  or1/1 -> Conv1/1
  ctrl_1L/8(output8) -> or8/4
  ctrl_1L/7(output7) -> or7/4
  ctrl_1L/6(output6) -> or6/4
  ctrl_1L/5(output5) -> or5/4
  ctrl_1L/4(output4) -> or4/4
  ctrl_1L/3(output3) -> or3/4
  ctrl_1L/2(output2) -> or2/4
  ctrl_1L/1(output1) -> or1/4
  max_n/8(output8) -> or8/3
  max_n/7(output7) -> or7/3
  max_n/6(output6) -> or6/3
  max_n/5(output5) -> or5/3
  max_n/4(output4) -> or4/3
  max_n/3(output3) -> or3/3
  max_n/2(output2) -> or2/3
  max_n/1(output1) -> or1/3
  TP_1L/8(output8) -> or8/2
  TP_1L/7(output7) -> or7/2
  TP_1L/6(output6) -> or6/2
  TP_1L/5(output5) -> or5/2
  TP_1L/4(output4) -> or4/2
  TP_1L/3(output3) -> or3/2
  TP_1L/2(output2) -> or2/2
  TP_1L/1(output1) -> or1/2
  TN_1L/8(output8) -> or8/1
  TN_1L/7(output7) -> or7/1
  TN_1L/6(output6) -> or6/1
  TN_1L/5(output5) -> or5/1
  TN_1L/4(output4) -> or4/1
  TN_1L/3(output3) -> or3/1
  TN_1L/2(output2) -> or2/1
  TN_1L/1(output1) -> or1/1
  ECU_1L_mux/1 -> output/1

== system 21-E/run/ctrl/ECU_1R ==
  TN_1R_in : Inport
  TP_1R_in : Inport  Port=2
  max_n_in : Inport  Port=3
  ctrl_1R_in : Inport  Port=4
  Conv{1..8} (8 alike) : DataTypeConversion
  ECU_1R_DLC : Constant  Value=8  OutDataTypeStr=uint8
  ECU_1R_DLC_Out : Terminator
  ECU_1R_ID : Constant  Value=389  OutDataTypeStr=single
  ECU_1R_ID_Out : Terminator
  ECU_1R_mux : Mux  Inputs=8
  TN_1R : Subsystem
  TP_1R : Subsystem
  ctrl_1R : Subsystem
  max_n : Subsystem
  or{1..8} (8 alike) : simulink/Logic and Bit Operations/Bitwise Operator  logicop=OR  UseBitMask=off  NumInputPorts=4  BitMask=bin2dec('11011001')  BitMaskRealWorld=Stored Integer
  output : Outport
  wires:
  ctrl_1R_in/1 -> ctrl_1R/1(ctrl_1R)
  max_n_in/1 -> max_n/1(max_n)
  TP_1R_in/1 -> TP_1R/1(TP_1R)
  TN_1R_in/1 -> TN_1R/1(TN_1R)
  ECU_1R_DLC/1 -> ECU_1R_DLC_Out/1
  ECU_1R_ID/1 -> ECU_1R_ID_Out/1
  Conv8/1 -> ECU_1R_mux/8
  or8/1 -> Conv8/1
  Conv7/1 -> ECU_1R_mux/7
  or7/1 -> Conv7/1
  Conv6/1 -> ECU_1R_mux/6
  or6/1 -> Conv6/1
  Conv5/1 -> ECU_1R_mux/5
  or5/1 -> Conv5/1
  Conv4/1 -> ECU_1R_mux/4
  or4/1 -> Conv4/1
  Conv3/1 -> ECU_1R_mux/3
  or3/1 -> Conv3/1
  Conv2/1 -> ECU_1R_mux/2
  or2/1 -> Conv2/1
  Conv1/1 -> ECU_1R_mux/1
  or1/1 -> Conv1/1
  ctrl_1R/8(output8) -> or8/4
  ctrl_1R/7(output7) -> or7/4
  ctrl_1R/6(output6) -> or6/4
  ctrl_1R/5(output5) -> or5/4
  ctrl_1R/4(output4) -> or4/4
  ctrl_1R/3(output3) -> or3/4
  ctrl_1R/2(output2) -> or2/4
  ctrl_1R/1(output1) -> or1/4
  max_n/8(output8) -> or8/3
  max_n/7(output7) -> or7/3
  max_n/6(output6) -> or6/3
  max_n/5(output5) -> or5/3
  max_n/4(output4) -> or4/3
  max_n/3(output3) -> or3/3
  max_n/2(output2) -> or2/3
  max_n/1(output1) -> or1/3
  TP_1R/8(output8) -> or8/2
  TP_1R/7(output7) -> or7/2
  TP_1R/6(output6) -> or6/2
  TP_1R/5(output5) -> or5/2
  TP_1R/4(output4) -> or4/2
  TP_1R/3(output3) -> or3/2
  TP_1R/2(output2) -> or2/2
  TP_1R/1(output1) -> or1/2
  TN_1R/8(output8) -> or8/1
  TN_1R/7(output7) -> or7/1
  TN_1R/6(output6) -> or6/1
  TN_1R/5(output5) -> or5/1
  TN_1R/4(output4) -> or4/1
  TN_1R/3(output3) -> or3/1
  TN_1R/2(output2) -> or2/1
  TN_1R/1(output1) -> or1/1
  ECU_1R_mux/1 -> output/1

== system 21-E/run/ctrl/ECU_2L ==
  TN_2L_in : Inport
  TP_2L_in : Inport  Port=2
  max_n_in : Inport  Port=3
  ctrl_2L_in : Inport  Port=4
  Conv{1..8} (8 alike) : DataTypeConversion
  ECU_2L_DLC : Constant  Value=8  OutDataTypeStr=uint8
  ECU_2L_DLC_Out : Terminator
  ECU_2L_ID : Constant  Value=392  OutDataTypeStr=single
  ECU_2L_ID_Out : Terminator
  ECU_2L_mux : Mux  Inputs=8
  TN_2L : Subsystem
  TP_2L : Subsystem
  ctrl_2L : Subsystem
  max_n : Subsystem
  or{1..8} (8 alike) : simulink/Logic and Bit Operations/Bitwise Operator  logicop=OR  UseBitMask=off  NumInputPorts=4  BitMask=bin2dec('11011001')  BitMaskRealWorld=Stored Integer
  output : Outport
  wires:
  ctrl_2L_in/1 -> ctrl_2L/1(ctrl_2L)
  max_n_in/1 -> max_n/1(max_n)
  TP_2L_in/1 -> TP_2L/1(TP_2L)
  TN_2L_in/1 -> TN_2L/1(TN_2L)
  ECU_2L_DLC/1 -> ECU_2L_DLC_Out/1
  ECU_2L_ID/1 -> ECU_2L_ID_Out/1
  Conv8/1 -> ECU_2L_mux/8
  or8/1 -> Conv8/1
  Conv7/1 -> ECU_2L_mux/7
  or7/1 -> Conv7/1
  Conv6/1 -> ECU_2L_mux/6
  or6/1 -> Conv6/1
  Conv5/1 -> ECU_2L_mux/5
  or5/1 -> Conv5/1
  Conv4/1 -> ECU_2L_mux/4
  or4/1 -> Conv4/1
  Conv3/1 -> ECU_2L_mux/3
  or3/1 -> Conv3/1
  Conv2/1 -> ECU_2L_mux/2
  or2/1 -> Conv2/1
  Conv1/1 -> ECU_2L_mux/1
  or1/1 -> Conv1/1
  ctrl_2L/8(output8) -> or8/4
  ctrl_2L/7(output7) -> or7/4
  ctrl_2L/6(output6) -> or6/4
  ctrl_2L/5(output5) -> or5/4
  ctrl_2L/4(output4) -> or4/4
  ctrl_2L/3(output3) -> or3/4
  ctrl_2L/2(output2) -> or2/4
  ctrl_2L/1(output1) -> or1/4
  max_n/8(output8) -> or8/3
  max_n/7(output7) -> or7/3
  max_n/6(output6) -> or6/3
  max_n/5(output5) -> or5/3
  max_n/4(output4) -> or4/3
  max_n/3(output3) -> or3/3
  max_n/2(output2) -> or2/3
  max_n/1(output1) -> or1/3
  TP_2L/8(output8) -> or8/2
  TP_2L/7(output7) -> or7/2
  TP_2L/6(output6) -> or6/2
  TP_2L/5(output5) -> or5/2
  TP_2L/4(output4) -> or4/2
  TP_2L/3(output3) -> or3/2
  TP_2L/2(output2) -> or2/2
  TP_2L/1(output1) -> or1/2
  TN_2L/8(output8) -> or8/1
  TN_2L/7(output7) -> or7/1
  TN_2L/6(output6) -> or6/1
  TN_2L/5(output5) -> or5/1
  TN_2L/4(output4) -> or4/1
  TN_2L/3(output3) -> or3/1
  TN_2L/2(output2) -> or2/1
  TN_2L/1(output1) -> or1/1
  ECU_2L_mux/1 -> output/1

== system 21-E/run/ctrl/ECU_2R ==
  TN_2R_in : Inport
  TP_2R_in : Inport  Port=2
  max_n_in : Inport  Port=3
  ctrl_2R_in : Inport  Port=4
  Conv{1..8} (8 alike) : DataTypeConversion
  ECU_2R_DLC : Constant  Value=8  OutDataTypeStr=uint8
  ECU_2R_DLC_Out : Terminator
  ECU_2R_ID : Constant  Value=393  OutDataTypeStr=single
  ECU_2R_ID_Out : Terminator
  ECU_2R_mux : Mux  Inputs=8
  TN_2R : Subsystem
  TP_2R : Subsystem
  ctrl_2R : Subsystem
  max_n : Subsystem
  or{1..8} (8 alike) : simulink/Logic and Bit Operations/Bitwise Operator  logicop=OR  UseBitMask=off  NumInputPorts=4  BitMask=bin2dec('11011001')  BitMaskRealWorld=Stored Integer
  output : Outport
  wires:
  ctrl_2R_in/1 -> ctrl_2R/1(ctrl_2R)
  max_n_in/1 -> max_n/1(max_n)
  TP_2R_in/1 -> TP_2R/1(TP_2R)
  TN_2R_in/1 -> TN_2R/1(TN_2R)
  ECU_2R_DLC/1 -> ECU_2R_DLC_Out/1
  ECU_2R_ID/1 -> ECU_2R_ID_Out/1
  Conv8/1 -> ECU_2R_mux/8
  or8/1 -> Conv8/1
  Conv7/1 -> ECU_2R_mux/7
  or7/1 -> Conv7/1
  Conv6/1 -> ECU_2R_mux/6
  or6/1 -> Conv6/1
  Conv5/1 -> ECU_2R_mux/5
  or5/1 -> Conv5/1
  Conv4/1 -> ECU_2R_mux/4
  or4/1 -> Conv4/1
  Conv3/1 -> ECU_2R_mux/3
  or3/1 -> Conv3/1
  Conv2/1 -> ECU_2R_mux/2
  or2/1 -> Conv2/1
  Conv1/1 -> ECU_2R_mux/1
  or1/1 -> Conv1/1
  ctrl_2R/8(output8) -> or8/4
  ctrl_2R/7(output7) -> or7/4
  ctrl_2R/6(output6) -> or6/4
  ctrl_2R/5(output5) -> or5/4
  ctrl_2R/4(output4) -> or4/4
  ctrl_2R/3(output3) -> or3/4
  ctrl_2R/2(output2) -> or2/4
  ctrl_2R/1(output1) -> or1/4
  max_n/8(output8) -> or8/3
  max_n/7(output7) -> or7/3
  max_n/6(output6) -> or6/3
  max_n/5(output5) -> or5/3
  max_n/4(output4) -> or4/3
  max_n/3(output3) -> or3/3
  max_n/2(output2) -> or2/3
  max_n/1(output1) -> or1/3
  TP_2R/8(output8) -> or8/2
  TP_2R/7(output7) -> or7/2
  TP_2R/6(output6) -> or6/2
  TP_2R/5(output5) -> or5/2
  TP_2R/4(output4) -> or4/2
  TP_2R/3(output3) -> or3/2
  TP_2R/2(output2) -> or2/2
  TP_2R/1(output1) -> or1/2
  TN_2R/8(output8) -> or8/1
  TN_2R/7(output7) -> or7/1
  TN_2R/6(output6) -> or6/1
  TN_2R/5(output5) -> or5/1
  TN_2R/4(output4) -> or4/1
  TN_2R/3(output3) -> or3/1
  TN_2R/2(output2) -> or2/1
  TN_2R/1(output1) -> or1/1
  ECU_2R_mux/1 -> output/1

== system 21-E/run/ctrl/Subsystem ==
  bre : Inport
  TN1L : Inport  Port=2
  TN1R : Inport  Port=3
  TN2L : Inport  Port=4
  TN2R : Inport  Port=5
  Data Store Read3 : DataStoreRead  DataStoreName=Vture
  Data Type Conversion2 : DataTypeConversion  OutDataTypeStr=double
  Demux : Demux
  Gain : Gain  Gain=-1
  Gain1 : Gain  Gain=1/0.0098
  Gain3 : Gain  Gain=1/12.5
  MATLAB Function : MATLAB Function  TreatAsAtomicUnit=on
  Mux : Mux
  Product : Product
  Subsystem : Subsystem
  N1L : Outport
  N1R : Outport  Port=2
  N2L : Outport  Port=3
  N2R : Outport  Port=4
  reg : Outport  Port=5
  wires:
  bre/1 -> MATLAB Function/2(bre)
  Data Store Read3/1 -> MATLAB Function/1(v)
  Gain3/1 -> Gain1/1
  Gain1/1 -> Data Type Conversion2/1
  Data Type Conversion2/1 -> Subsystem/1(In1)
  TN2L/1 -> Mux/3
  TN1R/1 -> Mux/2
  TN1L/1 -> Mux/1
  TN2R/1 -> Mux/4
  Mux/1 -> Gain3/1
  Subsystem/1(Out1) -> Product/2
  MATLAB Function/1(reg) -> Product/1, reg/1
  Product/1 -> Gain/1
  Gain/1 -> Demux/1
  Demux/1 -> N1L/1
  Demux/2 -> N1R/1
  Demux/3 -> N2L/1
  Demux/4 -> N2R/1

== system 21-E/run/ctrl/Subsystem1 ==
  acc : Inport
  reg : Inport  Port=2
  Add : Sum
  Add1 : Sum
  Constant : Constant
  Constant1 : Constant  Value=100
  Constant2 : Constant  Value=100
  Constant3 : Constant  Value=0.1
  Demux : Demux  Outputs=2
  Demux1 : Demux  Outputs=2
  ECCalVar : Constant  InitFcn=ecucoder_acal;  Value=add_k1_100  OutDataTypeStr=Inherit: Inherit via back propagation  SampleTime=-1
  ECCalVar2 : Constant  InitFcn=ecucoder_acal;  Value=add_k2_100  OutDataTypeStr=Inherit: Inherit via back propagation  SampleTime=-1
  Mux : Mux  Inputs=2
  Product : Product  Inputs=*/
  Product1 : Product  Inputs=*/
  Product2 : Product
  Product3 : Product
  Product4 : Product
  Saturation4 : Saturate  UpperLimit=1  LowerLimit=0
  Subsystem : Subsystem
  Sum : Sum  Inputs=|-+
  control : Subsystem
  TF : Outport
  TR : Outport  Port=2
  wires:
  Demux/1 -> Product2/2
  Constant3/1 -> Add1/1, Add/2
  Demux/2 -> Product3/2
  control/2(T2) -> Subsystem/2(T2d)
  Subsystem/1(T) -> Demux/1
  Saturation4/1 -> Product3/1, Product2/1
  control/1(T1) -> Subsystem/1(T1d)
  Product3/1 -> Mux/2  "T2"
  acc/1 -> Saturation4/1
  Product2/1 -> Mux/1  "T1"
  Constant1/1 -> Product/2
  ECCalVar2/1 -> Product1/1
  Product1/1 -> Add1/2
  ECCalVar/1 -> Product/1
  Add/1 -> control/1(k1)  "k1"
  Constant2/1 -> Product1/2
  Add1/1 -> control/2(k2)  "k2"
  Product/1 -> Add/1
  Constant/1 -> Product4/2, Sum/2
  Mux/1 -> Product4/1
  Product4/1 -> Demux1/1
  Demux1/1 -> TF/1
  Demux1/2 -> TR/1

== system 21-E/run/ctrl/Subsystem2 ==
  T1d : Inport
  T2d : Inport  Port=2
  Constant : Constant  Value=0.5
  Constant1 : Constant  Value=0.5
  Data Store Read1 : DataStoreRead  DataStoreName=Vture
  Data Store Read2 : DataStoreRead  DataStoreName=acc_signal
  Data Store Read3 : DataStoreRead  DataStoreName=Vture
  Data Type Conversion2 : DataTypeConversion  OutDataTypeStr=double
  Data Type Conversion3 : DataTypeConversion  OutDataTypeStr=double
  Gain : Gain  Gain=0.5
  Gain1 : Gain  Gain=1/0.0098
  Gain2 : Gain  Gain=1/0.0098
  Gain3 : Gain  Gain=1/12.5
  Gain4 : Gain  Gain=1/12.5
  Logical Operator : Logic  AllPortsSameDT=off  OutDataTypeStr=boolean
  MATLAB Function : MATLAB Function  TreatAsAtomicUnit=on
  Mux : Mux  Inputs=2
  Relational Operator : RelationalOperator  Operator=>  OutDataTypeStr=boolean
  Relational Operator1 : RelationalOperator  Operator=<=  OutDataTypeStr=boolean
  Subsystem : Subsystem
  Subsystem1 : Subsystem
  Switch : Switch  Criteria=u2 > Threshold
  T : Outport
  wires:
  Gain3/1 -> Gain1/1
  T1d/1 -> Gain3/1
  Gain2/1 -> Data Type Conversion3/1
  Gain1/1 -> Data Type Conversion2/1
  T2d/1 -> Gain4/1
  Gain4/1 -> Gain2/1
  Data Type Conversion2/1 -> Subsystem/1(In1)
  Data Type Conversion3/1 -> Subsystem1/1(In1)
  Data Store Read1/1 -> MATLAB Function/1(v)
  Subsystem/1(Out1) -> MATLAB Function/2(T1d)
  Subsystem1/1(Out1) -> MATLAB Function/3(T2d)
  Data Store Read2/1 -> Relational Operator/1
  Constant/1 -> Relational Operator/2
  Relational Operator/1 -> Logical Operator/1
  Data Store Read3/1 -> Relational Operator1/1
  Constant1/1 -> Relational Operator1/2
  Relational Operator1/1 -> Logical Operator/2
  Logical Operator/1 -> Switch/2
  MATLAB Function/1(T1) -> Mux/1
  MATLAB Function/2(T2) -> Mux/2
  Mux/1 -> Switch/3, Gain/1
  Gain/1 -> Switch/1
  Switch/1 -> T/1

== system 21-E/run/ctrl/amk_tpostive1 ==
  acc_signal : Inport
  Data Store Read1 : DataStoreRead  DataStoreName=Vture
  Data Type Conversion : DataTypeConversion  OutMin=[0]  OutMax=[1]  OutDataTypeStr=double
  Divide1 : Product  Inputs=**  OutDataTypeStr=uint16
  MATLAB Function : MATLAB Function  TreatAsAtomicUnit=on
  Saturation3 : Saturate  UpperLimit=2100  LowerLimit=0
  Saturation4 : Saturate  UpperLimit=1  LowerLimit=0
  工况判断 : Subsystem  Commented=on
  差速 : Subsystem  Commented=on
  限滑 : Subsystem
  1L : Outport
  1R : Outport  Port=2
  2L : Outport  Port=3
  2R : Outport  Port=4
  wires:
  MATLAB Function/1(T) -> Saturation3/1
  Saturation3/1 -> Divide1/1
  Saturation4/1 -> Divide1/2
  Data Type Conversion/1 -> Saturation4/1
  acc_signal/1 -> Data Type Conversion/1
  差速/4(Out4) -> 工况判断/8(In8)
  差速/3(Out3) -> 工况判断/7(In7)
  差速/2(Out2) -> 工况判断/6(In6)
  差速/1(Out1) -> 工况判断/5(In5)
  Data Store Read1/1 -> MATLAB Function/1(v)
  Divide1/1 -> 限滑/1(TP)
  限滑/4(Out4) -> 2R/1
  限滑/3(Out3) -> 2L/1
  限滑/2(Out2) -> 1R/1
  限滑/1(Out1) -> 1L/1

== system 21-E/run/ctrl/control ==
  k1 : Inport
  k2 : Inport  Port=2
  Data Store Write : DataStoreWrite  DataStoreName=slip_qian
  Data Store Write1 : DataStoreWrite  DataStoreName=slip_hou
  Subsystem : Subsystem
  Subsystem1 : Subsystem
  Subsystem2 : Subsystem
  Subsystem3 : Subsystem
  Subsystem4 : Subsystem
  Subsystem5 : Subsystem
  Subsystem6 : Subsystem
  T1 : Outport
  T2 : Outport  Port=2
  wires:
  Subsystem6/2(alp2d) -> [alp2]
  Subsystem/2(x2) -> [x2], Subsystem1/2(x2)
  Subsystem/1(x1) -> [x1], Subsystem1/1(x1)
  Subsystem/3(x3) -> Subsystem1/3(v)
  [phy1] -> Subsystem4/1(phy1)
  [alp1] -> Subsystem4/2(alp1)
  Subsystem6/1(alp1d) -> [alp1]
  Subsystem4/1(T1) -> T1/1
  k1/1 -> Subsystem6/5(k1)
  Subsystem3/1(W1) -> [w1]
  [phy2] -> Subsystem5/1(phy2)
  Subsystem2/2(phy2) -> [phy2]
  [x2] -> Subsystem6/2(x2)
  Subsystem3/2(W2) -> [w2]
  Subsystem2/1(phy1) -> [phy1]
  [x1] -> Subsystem6/1(x1)
  Subsystem1/2(s2) -> Data Store Write1/1, Subsystem2/2(s2)
  k2/1 -> Subsystem6/6(k2)
  Subsystem1/4(x4) -> Subsystem6/4(x4)
  Subsystem1/1(s1) -> Data Store Write/1, Subsystem2/1(s1)
  Subsystem1/3(x3) -> Subsystem6/3(x3)
  [alp2] -> Subsystem5/2(alp2)
  Subsystem5/1(T2) -> T2/1
  [w2] -> Subsystem5/3(W2)
  [w1] -> Subsystem4/3(W1)
  [phy1] -> Subsystem3/1(phy1)
  [phy2] -> Subsystem3/2(phy2)

== system 21-E/run/ctrl/ECU_1L/TN_1L ==
  TN_1L : Inport
  BitCov : DataTypeConversion  OutDataTypeStr=uint8
  Constant{1..6} (6 alike) : Constant  Value=0  OutDataTypeStr=uint8
  TN_1LABS : Abs
  TN_1LCOV : DataTypeConversion  OutDataTypeStr=uint8
  TN_1LCS : ArithShift  BitShiftNumber=-16
  TN_1LConS : Constant  OutDataTypeStr=single
  TN_1LCosR : Constant  Value=0  OutDataTypeStr=uint8
  TN_1LROP : RelationalOperator  Operator=<  OutDataTypeStr=boolean
  TN_1LRon : Rounding  Operator=round
  TN_1LSW : Switch  Criteria=u2 ~= 0
  TN_1L_1sat : Saturate  UpperLimit=65535  LowerLimit=0
  TN_1L_And : simulink/Logic and Bit Operations/Bitwise Operator  logicop=AND  UseBitMask=off  NumInputPorts=2  BitMask=bin2dec('11011001')  BitMaskRealWorld=Stored Integer
  TN_1L_And_C : Constant  Value=255  OutDataTypeStr=uint32
  TN_1L_Convert : DataTypeConversion  OutDataTypeStr=uint32
  TN_1L_D : Product  Inputs=*/
  TN_1L_D1 : Product  Inputs=*/
  TN_1L_F : Constant  OutDataTypeStr=single
  TN_1L_L : simulink/Logic and Bit Operations/Bitwise Operator  logicop=AND  UseBitMask=on  BitMask=65535  BitMaskRealWorld=Stored Integer
  TN_1L_O : Constant  Value=0  OutDataTypeStr=single
  TN_1L_S : ArithShift
  TN_1L_sat : Saturate  UpperLimit=32767  LowerLimit=-32768
  TN_1L_st : Sum  Inputs=+-
  TN_1Loutput8_C : Constant  Value=256
  TN_1Lsubcon : Sum  Inputs=+-
  output1 : Outport
  output2 : Outport  Port=2
  output3 : Outport  Port=3
  output4 : Outport  Port=4
  output5 : Outport  Port=5
  output6 : Outport  Port=6
  output7 : Outport  Port=7
  output8 : Outport  Port=8
  wires:
  Constant6/1 -> output6/1
  Constant5/1 -> output5/1
  Constant4/1 -> output4/1
  Constant3/1 -> output3/1
  Constant2/1 -> output2/1
  Constant1/1 -> output1/1
  BitCov/1 -> output7/1
  TN_1L_And/1 -> BitCov/1
  TN_1L_And_C/1 -> TN_1L_And/2
  TN_1LCOV/1 -> output8/1
  TN_1L_D1/1 -> TN_1LCOV/1
  TN_1Loutput8_C/1 -> TN_1L_D1/2
  TN_1L_L/1 -> TN_1L_And/1, TN_1L_D1/1
  TN_1L_Convert/1 -> TN_1L_L/1
  TN_1L_1sat/1 -> TN_1L_Convert/1
  TN_1L_S/1 -> TN_1L_1sat/1
  TN_1LSW/1 -> TN_1L_S/1
  TN_1LROP/1 -> TN_1LSW/2
  TN_1Lsubcon/1 -> TN_1LSW/1
  TN_1LABS/1 -> TN_1Lsubcon/2
  TN_1LCS/1 -> TN_1Lsubcon/1
  TN_1LConS/1 -> TN_1LCS/1
  TN_1LCosR/1 -> TN_1LROP/2
  TN_1LRon/1 -> TN_1LSW/3, TN_1LABS/1, TN_1LROP/1
  TN_1L_D/1 -> TN_1LRon/1
  TN_1L_F/1 -> TN_1L_D/2
  TN_1L_st/1 -> TN_1L_D/1
  TN_1L_O/1 -> TN_1L_st/2
  TN_1L_sat/1 -> TN_1L_st/1
  TN_1L/1 -> TN_1L_sat/1

== system 21-E/run/ctrl/ECU_1L/TP_1L ==
  TP_1L : Inport
  BitCov : DataTypeConversion  OutDataTypeStr=uint8
  Constant{1..4,7..8} (6 alike) : Constant  Value=0  OutDataTypeStr=uint8
  TP_1LABS : Abs
  TP_1LCOV : DataTypeConversion  OutDataTypeStr=uint8
  TP_1LCS : ArithShift  BitShiftNumber=-16
  TP_1LConS : Constant  OutDataTypeStr=single
  TP_1LCosR : Constant  Value=0  OutDataTypeStr=uint8
  TP_1LROP : RelationalOperator  Operator=<  OutDataTypeStr=boolean
  TP_1LRon : Rounding  Operator=round
  TP_1LSW : Switch  Criteria=u2 ~= 0
  TP_1L_1sat : Saturate  UpperLimit=65535  LowerLimit=0
  TP_1L_And : simulink/Logic and Bit Operations/Bitwise Operator  logicop=AND  UseBitMask=off  NumInputPorts=2  BitMask=bin2dec('11011001')  BitMaskRealWorld=Stored Integer
  TP_1L_And_C : Constant  Value=255  OutDataTypeStr=uint32
  TP_1L_Convert : DataTypeConversion  OutDataTypeStr=uint32
  TP_1L_D : Product  Inputs=*/
  TP_1L_D1 : Product  Inputs=*/
  TP_1L_F : Constant  OutDataTypeStr=single
  TP_1L_L : simulink/Logic and Bit Operations/Bitwise Operator  logicop=AND  UseBitMask=on  BitMask=65535  BitMaskRealWorld=Stored Integer
  TP_1L_O : Constant  Value=0  OutDataTypeStr=single
  TP_1L_S : ArithShift
  TP_1L_sat : Saturate  UpperLimit=32767  LowerLimit=-32768
  TP_1L_st : Sum  Inputs=+-
  TP_1Loutput6_C : Constant  Value=256
  TP_1Lsubcon : Sum  Inputs=+-
  output1 : Outport
  output2 : Outport  Port=2
  output3 : Outport  Port=3
  output4 : Outport  Port=4
  output5 : Outport  Port=5
  output6 : Outport  Port=6
  output7 : Outport  Port=7
  output8 : Outport  Port=8
  wires:
  Constant8/1 -> output8/1
  Constant7/1 -> output7/1
  Constant4/1 -> output4/1
  Constant3/1 -> output3/1
  Constant2/1 -> output2/1
  Constant1/1 -> output1/1
  BitCov/1 -> output5/1
  TP_1L_And/1 -> BitCov/1
  TP_1L_And_C/1 -> TP_1L_And/2
  TP_1LCOV/1 -> output6/1
  TP_1L_D1/1 -> TP_1LCOV/1
  TP_1Loutput6_C/1 -> TP_1L_D1/2
  TP_1L_L/1 -> TP_1L_And/1, TP_1L_D1/1
  TP_1L_Convert/1 -> TP_1L_L/1
  TP_1L_1sat/1 -> TP_1L_Convert/1
  TP_1L_S/1 -> TP_1L_1sat/1
  TP_1LSW/1 -> TP_1L_S/1
  TP_1LROP/1 -> TP_1LSW/2
  TP_1Lsubcon/1 -> TP_1LSW/1
  TP_1LABS/1 -> TP_1Lsubcon/2
  TP_1LCS/1 -> TP_1Lsubcon/1
  TP_1LConS/1 -> TP_1LCS/1
  TP_1LCosR/1 -> TP_1LROP/2
  TP_1LRon/1 -> TP_1LSW/3, TP_1LABS/1, TP_1LROP/1
  TP_1L_D/1 -> TP_1LRon/1
  TP_1L_F/1 -> TP_1L_D/2
  TP_1L_st/1 -> TP_1L_D/1
  TP_1L_O/1 -> TP_1L_st/2
  TP_1L_sat/1 -> TP_1L_st/1
  TP_1L/1 -> TP_1L_sat/1
